simulink model "Example1"  (Simulink 8.8)
settings: Solver=FixedStepDiscrete  StartTime=0.0  StopTime=10.0  FixedStep=0.0003125  RelTol=1e-3  EnableMultiTasking=on
settings Model: Creator=monika  LastModifiedBy=monika
settings OptimizationCC: ExpressionDepthLimit=2147483647  LifeSpan=1
settings DebuggingCC: CheckSSInitialOutputMsg=off  SolverPrmCheckMsg=warning
settings RTWCC: SystemTargetFile=ert.tlc  TemplateMakefile=ert_default_tmf  Description=Embedded Coder
settings CodeAppCC: IgnoreCustomStorageClasses=off  CustomSymbolStrType=$N$R$M  InternalIdentifier=Classic
settings ERTTargetCC: MultiwordLength=2048  GenerateSampleERTMain=on  ERTCustomFileTemplate=example_file_process.tlc  ConvertIfToSwitch=off  SuppressUnreachableDefaultCases=off

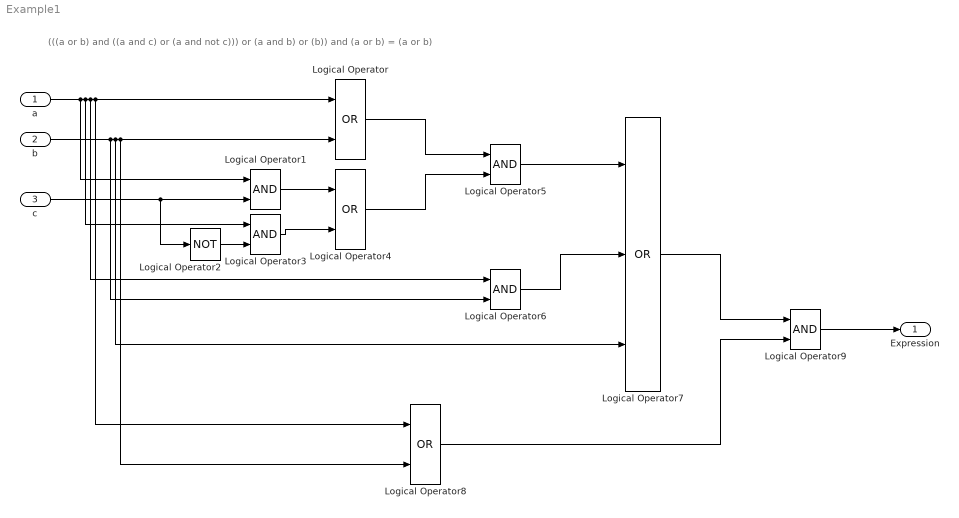
== system Example1 ==
  note: (((a or b) and ((a and c) or (a and not c))) or (a and b) or (b)) and (a or b) = (a or b)
  a : Inport
  b : Inport  Port=2
  c : Inport  Port=3
  Logical Operator : Logic  Operator=OR  AllPortsSameDT=off  OutDataTypeStr=boolean
  Logical Operator{1,3,5..6,9} (5 alike) : Logic  AllPortsSameDT=off  OutDataTypeStr=boolean
  Logical Operator2 : Logic  Operator=NOT  AllPortsSameDT=off  OutDataTypeStr=boolean
  Logical Operator4 : Logic  Operator=OR  AllPortsSameDT=off  OutDataTypeStr=boolean
  Logical Operator7 : Logic  Operator=OR  Inputs=3  AllPortsSameDT=off  OutDataTypeStr=boolean
  Logical Operator8 : Logic  Operator=OR  AllPortsSameDT=off  OutDataTypeStr=boolean
  Expression : Outport
  wires:
  Logical Operator2/1 -> Logical Operator3/2
  Logical Operator1/1 -> Logical Operator4/1
  Logical Operator3/1 -> Logical Operator4/2
  Logical Operator/1 -> Logical Operator5/1
  Logical Operator4/1 -> Logical Operator5/2
  Logical Operator5/1 -> Logical Operator7/1
  Logical Operator6/1 -> Logical Operator7/2
  c/1 -> Logical Operator2/1, Logical Operator1/2
  Logical Operator9/1 -> Expression/1
  Logical Operator7/1 -> Logical Operator9/1
  Logical Operator8/1 -> Logical Operator9/2
  a/1 -> Logical Operator1/1, Logical Operator3/1, Logical Operator6/1, Logical Operator/1, Logical Operator8/1
  b/1 -> Logical Operator6/2, Logical Operator7/3, Logical Operator/2, Logical Operator8/2
